simulink model "constrained_second_link"  (R2020b)
settings: Solver=VariableStepAuto  StartTime=0.0  StopTime=100.0  RelTol=1e-3
values from neighbouring files (symbols this model uses):
  b1 = 5.33518    [Linearization.m]    (also in MainScript_PID.m; calib_up_up.m; tune_parameters.m = 4.8; tune_parameters_cl.m)
  b2 = 4e-05    [Linearization.m]    (also in MainScript_PID.m; calib_up_up.m; tune_parameters.m = 5e-05; tune_parameters_cl.m = 3.7644e-05)
  c1 = 0.01    [Linearization.m]    (also in MainScript_PID.m; calib_up_up.m; tune_parameters.m = -0.04; tune_parameters_cl.m = 0.025)
  c2 = 0.07    [Linearization.m]    (also in MainScript_PID.m; calib_up_up.m; tune_parameters.m = 0.0644; tune_parameters_cl.m = 0.0644)
  g = 9.81    [Linearization.m]    (also in MainScript_PID.m; calib_up_up.m; tune_parameters.m; tune_parameters_cl.m)
  I1 = 0.01076    [Linearization.m]    (also in MainScript_PID.m; calib_up_up.m; tune_parameters.m = 0.074; tune_parameters_cl.m = 0.018544)
  I2 = 0.0001    [Linearization.m]    (also in MainScript_PID.m; calib_up_up.m; tune_parameters.m; tune_parameters_cl.m = 8.3382e-05)
  km = 39.2954    [Linearization.m]    (also in MainScript_PID.m = 42.2954; calib_up_up.m; tune_parameters.m = 50; tune_parameters_cl.m)
  l1 = 0.0897    [Linearization.m]    (also in MainScript_PID.m; calib_up_up.m; tune_parameters.m = 0.1; tune_parameters_cl.m)
  m1 = 0.2    [Linearization.m]    (also in MainScript_PID.m; calib_up_up.m; tune_parameters.m = 0.125; tune_parameters_cl.m = 0.53513)
  m2 = 0.087972    [Linearization.m]    (also in MainScript_PID.m; calib_up_up.m; tune_parameters.m = 0.0528; tune_parameters_cl.m = 0.0528)
  te = 0.01    [Linearization.m]    (also in MainScript_PID.m = 0.008; calib_up_up.m; tune_parameters.m = 0.03; tune_parameters_cl.m = 0.00258)
  theta0 = [-pi;3*pi/4]    [Compute_whitebox.m]    (also in MainScript_PID.m = [-pi;     pi/4]; calib_up_up.m = [0;-pi]; tune_parameters.m = [-pi;10*pi/12]; tune_parameters_cl.m = [-pi;-pi])
  thetadot0 = [0;0]    [MainScript_PID.m]    (also in calib_up_up.m; tune_parameters.m; tune_parameters_cl.m; tune_parameters_theta1.m)
settings Model: Creator=llaporte  LastModifiedBy=llaporte

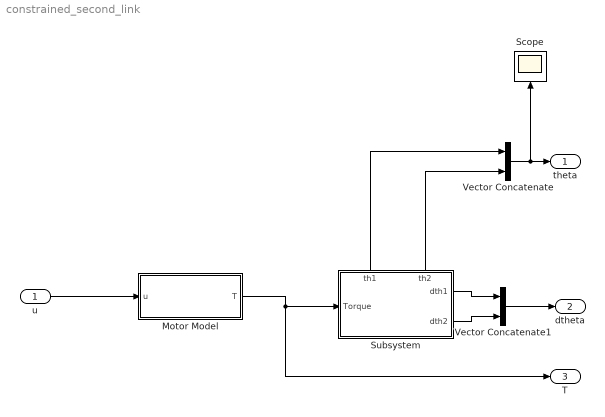
== system constrained_second_link ==
  u : Inport
  "Motor Model " : Subsystem
  Scope : Scope
  Subsystem : Subsystem
      settings: PortSchema="{\"entries\":[{\"content\":{\"sides\":[{\"content\":{\"connectorIds\":[\"In1\"]},\"type\":\"ConnectorPlacement.EquallySpacedRectSide\",\"uuid\":\"5594a261-93f1-4f8b-b3a7-645a5ddd664f\"},{\"content\":{\"connectorIds\":[\"Out1\",\"Out2\"],\"side\":\"RIGHT\"},\"type\":\"ConnectorPlacement.EquallySpacedRectSide\",\"uuid\":\"9901c30e-5b59-453a-a3bf-c77471a935d6\"},{\"content\":{\"connectorIds\":[\"Out3\",\"Out4\"],\"side\":\"TOP\"},\"type\":\"ConnectorPlacement.EquallySpacedRectSide\",\"uuid\":\"5fa97dcb-98b1-4f62-888a-f38643244b0a\"},{\"content\":{\"connectorIds\":[],\"side\":\"HIDDEN\"},\"type\":\"ConnectorPlacement.EquallySpacedRectSide\",\"uuid\":\"38d25c3a-e617-425c-94ac-957497bbff87\"}]},\"type\":\"ConnectorPlacement.EquallySpacedConnector\",\"uuid\":\"2121014f-6857-48e5-b99a-933752d348c5\"}],\"packageUris\":[\"http://schema.mathworks.com/mf0/Connector/R2020b\"],\"version\":\"1.0\"}"
  Vector Concatenate : Concatenate
  Vector Concatenate1 : Concatenate
  theta : Outport
  dtheta : Outport  Port=2
  T : Outport  Port=3
  wires:
  u/1 -> "Motor Model "/1(u)
  "Motor Model "/1(T) -> Subsystem/1(Torque), T/1
  Subsystem/3(th1) -> Vector Concatenate/1
  Vector Concatenate/1 -> Scope/1, theta/1
  Subsystem/1(dth1) -> Vector Concatenate1/1
  Subsystem/2(dth2) -> Vector Concatenate1/2
  Vector Concatenate1/1 -> dtheta/1
  Subsystem/4(th2) -> Vector Concatenate/2

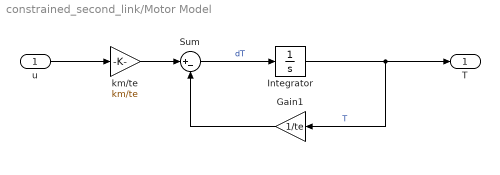
== system constrained_second_link/Motor Model  ==
  u : Inport
  Gain1 : Gain  Gain=1/te
  Integrator : Integrator
  Sum : Sum  Inputs=|+-
  "km/te " : Gain  Gain=km/te
  T : Outport
  wires:
  "km/te "/1 -> Sum/1
  u/1 -> "km/te "/1
  Integrator/1 -> T/1, Gain1/1  "T"
  Sum/1 -> Integrator/1  "dT"
  Gain1/1 -> Sum/2

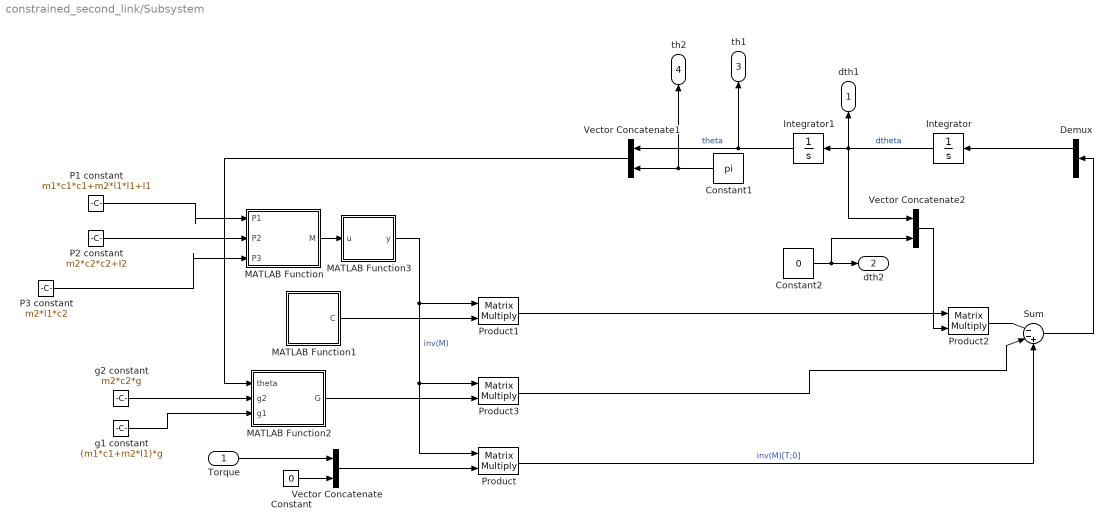
== system constrained_second_link/Subsystem ==
  Torque : Inport
  Constant : Constant  Value=0
  Constant1 : Constant  Value=pi
  Constant2 : Constant  Value=0
  Demux : Demux  Outputs=2
  Integrator : Integrator  InitialCondition=thetadot0(1)
  Integrator1 : Integrator  InitialCondition=theta0(1)
  MATLAB Function : MATLAB Function  TreatAsAtomicUnit=on
  MATLAB Function1 : MATLAB Function  TreatAsAtomicUnit=on
  MATLAB Function2 : MATLAB Function  TreatAsAtomicUnit=on
  MATLAB Function3 : MATLAB Function  TreatAsAtomicUnit=on
  P1 constant : Constant  Value=m1*c1*c1+m2*l1*l1+I1
  P2 constant : Constant  Value=m2*c2*c2+I2
  P3 constant : Constant  Value=m2*l1*c2
  Product{,1..3} (4 alike) : Product  Multiplication=Matrix(*)
  Sum : Sum  Inputs=|--+
  Vector Concatenate : Concatenate
  Vector Concatenate1 : Concatenate
  Vector Concatenate2 : Concatenate
  g1 constant : Constant  Value=(m1*c1+m2*l1)*g
  g2 constant : Constant  Value=m2*c2*g
  dth1 : Outport
  dth2 : Outport  Port=2
  th1 : Outport  Port=3
  th2 : Outport  Port=4
  wires:
  MATLAB Function2/1(G) -> Product3/2
  Product2/1 -> Sum/1
  g1 constant/1 -> MATLAB Function2/3(g1)
  P3 constant/1 -> MATLAB Function/3(P3)
  Torque/1 -> Vector Concatenate/1
  Vector Concatenate/1 -> Product/2
  Integrator/1 -> Integrator1/1, Vector Concatenate2/1, dth1/1  "dtheta"
  Constant/1 -> Vector Concatenate/2
  P2 constant/1 -> MATLAB Function/2(P2)
  MATLAB Function3/1(y) -> Product3/1, Product/1, Product1/1  "inv(M)"
  MATLAB Function1/1(C) -> Product1/2
  g2 constant/1 -> MATLAB Function2/2(g2)
  Product3/1 -> Sum/2
  MATLAB Function/1(M) -> MATLAB Function3/1(u)
  Product/1 -> Sum/3  "inv(M)[T;0]"
  Product1/1 -> Product2/1
  P1 constant/1 -> MATLAB Function/1(P1)
  Integrator1/1 -> Vector Concatenate1/1, th1/1  "theta"
  Vector Concatenate1/1 -> MATLAB Function2/1(theta)
  Constant1/1 -> Vector Concatenate1/2, th2/1
  Sum/1 -> Demux/1
  Constant2/1 -> Vector Concatenate2/2, dth2/1
  Vector Concatenate2/1 -> Product2/2
  Demux/1 -> Integrator/1

== matlab function constrained_second_link/Subsystem/MATLAB Function ==
  data: M output; P1 input; P2 input; P3 input
function M = M_matrix(P1, P2, P3)
    M = [P1+P2-2*P3 P2-P3;
         P2-P3      P2];

== matlab function constrained_second_link/Subsystem/MATLAB Function1 ==
  data: C output; b1 parameter; b2 parameter
function C = C_matrix(b1, b2)
C = [b1 0;
     0  b2];

== matlab function constrained_second_link/Subsystem/MATLAB Function2 ==
  data: theta input; G output; g2 input; g1 input
function G = G_matrix(theta,g2, g1)
G = [sin(theta(1))*(g2-g1);
     g2*sin(theta(1))];

== matlab function constrained_second_link/Subsystem/MATLAB Function3 ==
  data: u input; y output
function y = inverse(u)
y = inv(u);
